simulink model "simulink_simulation"  (R2021a)
settings: Solver=VariableStepAuto  StartTime=0.0  StopTime=20  RelTol=1e-3
libraries: SignalEditorBlockLib x1, checkpacklib x1
settings Model: Creator=vash  LastModifiedBy=thodkatz

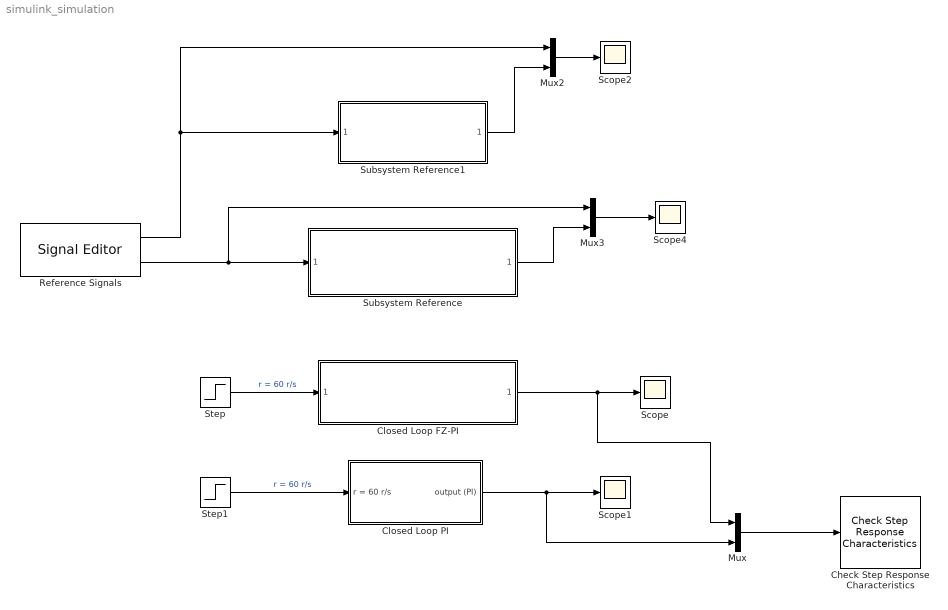
== system simulink_simulation ==
  " Reference Signals" : SignalEditorBlockLib/Signal Editor  FileName=customReferenceSignals.mat  ActiveScenario=Scenario  ActiveSignal=Squared  IsBus=off  OutputBusObjectStr=Bus: BusObject  SampleTime=0.01  Interpolate=off  ZeroCross=off  OutputAfterFinalValue=Setting to zero  Unit=inherit  PreserveSignalName=on
  Check Step Response Characteristics : checkpacklib/Check Step Response  Characteristics  InstantiateOnLoad=on  enabled=on  stopWhenAssertionFail=off  export=off  ViewDlgPos=[1 31 1920 973]  OpenViewOnLoad=off  LaunchViewOnOpen=on  TimeUnits=seconds  EnableStepResponseBound=on  InitialValue=0  FinalValue=60  StepTime=0  RiseTime=0.8  PercentRise=80  SettlingTime=9  PercentSettling=3  PercentOvershoot=7  PercentUndershoot=1
      settings: SourceProductBaseCode=CT,ID,MT,SO
  Closed Loop FZ-PI : Subsystem  ReferencedSubsystem=closedLoopFuzzyPI
  Closed Loop PI : Subsystem
  Mux : Mux  Inputs=2
  Mux2 : Mux  Inputs=2
  Mux3 : Mux  Inputs=2
  Scope{,1..2,4} (4 alike) : Scope
  Step : Step  Before=60  After=60  SampleTime=0.01
  Step1 : Step  Before=60  After=60  SampleTime=0.01
  Subsystem Reference : Subsystem  ReferencedSubsystem=closedLoopFuzzyPI
  Subsystem Reference1 : Subsystem  ReferencedSubsystem=closedLoopFuzzyPI
  wires:
  Closed Loop PI/1(output (PI)) -> Mux/2, Scope1/1
  Step1/1 -> Closed Loop PI/1(r = 60 r/s)  "r = 60 r/s"
  Step/1 -> Closed Loop FZ-PI/1  "r = 60 r/s"
  Mux3/1 -> Scope4/1
  Subsystem Reference/1 -> Mux3/2
  " Reference Signals"/2 -> Mux3/1, Subsystem Reference/1
  Closed Loop FZ-PI/1 -> Mux/1, Scope/1
  Mux/1 -> Check Step Response Characteristics/1
  Subsystem Reference1/1 -> Mux2/2
  Mux2/1 -> Scope2/1
  " Reference Signals"/1 -> Mux2/1, Subsystem Reference1/1

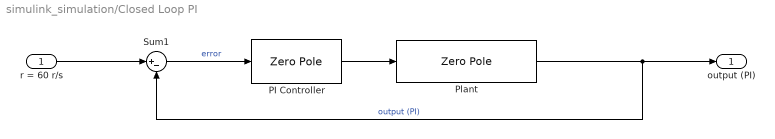
== system simulink_simulation/Closed Loop PI ==
  r = 60 r/s : Inport
  PI Controller : ZeroPole  Zeros=[-1.5]  Poles=[0]  Gain=1
  Plant : ZeroPole  Zeros=[]  Poles=[-1 -9]  Gain=10
  Sum1 : Sum  Inputs=|+-
  output (PI) : Outport
  wires:
  PI Controller/1 -> Plant/1
  Plant/1 -> Sum1/2, output (PI)/1  "output (PI)"
  r = 60 r/s/1 -> Sum1/1
  Sum1/1 -> PI Controller/1  "error"
